simulink model "model_car_unweighted"  (R2013b)
settings: Solver=ode45  StartTime=0.0  StopTime=2  FixedStep=0.001  RelTol=1e-3
libraries: cstblocks x5
settings Model: Creator=daniel  LastModifiedBy=daniel
settings ModelReferenceCC: ModelReferenceNumInstancesAllowed=Single

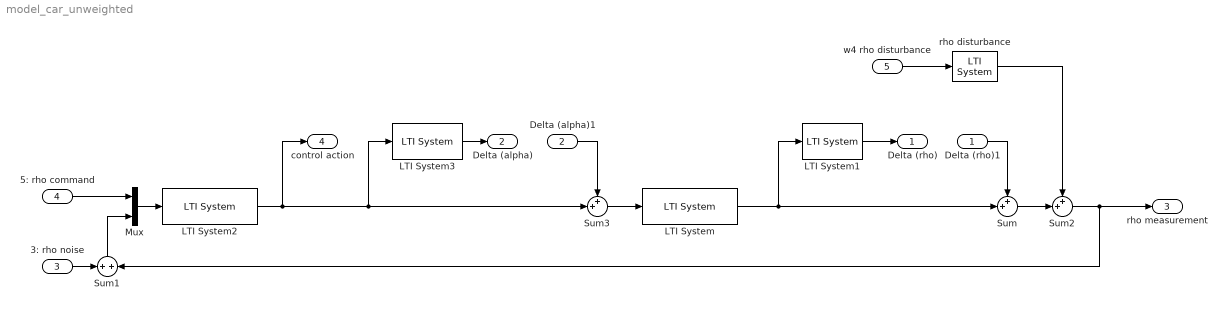
== system model_car_unweighted ==
  Delta (rho)1 : Inport
  Delta (alpha)1 : Inport  Port=2
  3: rho noise : Inport  Port=3
  5: rho command : Inport  Port=4
  w4 rho disturbance : Inport  Port=5
  LTI System : cstblocks/LTI System  sys=P_car  IC=[]
  LTI System1 : cstblocks/LTI System  sys=W_rho  IC=[]
  LTI System2 : cstblocks/LTI System  sys=K_sim  IC=[]
  LTI System3 : cstblocks/LTI System  sys=W_alpha  IC=[]
  Mux : Mux  Inputs=2
  Sum : Sum  Inputs=++|
  Sum1 : Sum
  Sum2 : Sum  Inputs=++|
  Sum3 : Sum  Inputs=++|
  rho disturbance : cstblocks/LTI System  sys=W_rhod  IC=[]
  Delta (rho) : Outport
  Delta (alpha) : Outport  Port=2
  rho measurement : Outport  Port=3
  control action : Outport  Port=4
  wires:
  LTI System/1 -> LTI System1/1, Sum/2
  LTI System1/1 -> Delta (rho)/1
  Delta (rho)1/1 -> Sum/1
  5: rho command/1 -> Mux/1
  3: rho noise/1 -> Sum1/1
  Sum2/1 -> Sum1/2, rho measurement/1
  w4 rho disturbance/1 -> rho disturbance/1
  rho disturbance/1 -> Sum2/1
  Sum/1 -> Sum2/2
  Mux/1 -> LTI System2/1
  Sum1/1 -> Mux/2
  LTI System2/1 -> LTI System3/1, Sum3/2, control action/1
  LTI System3/1 -> Delta (alpha)/1
  Delta (alpha)1/1 -> Sum3/1
  Sum3/1 -> LTI System/1
